simulink model "Australian14gen_forming_inertia"  (R2017b)
settings: Solver=ode23tb  StartTime=0.0  StopTime=100  FixedStep=1e-3  RelTol=1e-3  AbsTol=1e-3  EnableMultiTasking=on
PreLoadFcn:
  | dataaustralian14gen
values from neighbouring files (symbols this model uses):
  bus_v = [ 101	15 ... (first row only)    [dataaustralian14gen.m]
  c_fil = 1e-5*ones(15,1)    [dataaustralian14gen.m]
  comp = [ 1	211	0	0 ... (first row only)    [dataaustralian14gen.m]
  dist = sys.follin.dist    [main_following.m]    (also in main_forming.m = sys.formin.dist)
  Exc = [ 101	0	 200	0.1	    13.25  2.5	 0	0       0       0       0       0 ... (first row only)    [dataaustralian14gen.m]
  FH = 13    [dataaustralian14gen.m]
  FI = 1    [dataaustralian14gen.m]
  FL = .1    (= 0.1)    [dataaustralian14gen.m]
  G_data = [ 101	333.3	15	3.6	0.14	1.1	0.65	0.25	8.5     0.25	0.05	0       0       0.25	0.2 	0 ... (first row only)    [dataaustralian14gen.m]
  KH = 120    [dataaustralian14gen.m]
  KI = 10    [dataaustralian14gen.m]
  KL = 10    [dataaustralian14gen.m]
  Kvsc = 0*Kvsc    [dataaustralian14gen.m]    (also in optimgains.mat = [-4.89904313526 -21.043852985 -7.4754770322 -20.8245159401 -)
  l_fil = 5e-3*ones(15,1)    [dataaustralian14gen.m]
  line = [ 102	217	0.0084	0.0667	0.817	330	1 ... (first row only)    [dataaustralian14gen.m]
  load_mag = load_case4    [dataaustralian14gen.m]
  p = p_case4    [dataaustralian14gen.m]
  Pinit = [0.405553120017514,0.262363656270440,0.245287066765904,0.511573619715646,0.238910511748616,0.266289198874107,0.405451933295266,0.301363467877759,0.299904641553078,0.238601214125575,0.201576196829353,0.166515071179716,0.281316548159335,0.249279775700722,0.436119451429005]    [dataaustralian14gen.m]
  PSSMODEL = 1    [dataaustralian14gen.m]
  r_fil = 5e-1*ones(15,1)    [dataaustralian14gen.m]
  trans = [ 1	101	102	15	330	333.3	12	12 ... (first row only)    [dataaustralian14gen.m]
undefined symbols (not defined in the file or in its folder): D1, Delta, sys, thetavsc0
libraries: powerlib x399, Library x15, sps_avr x10, powerlib_extras x5
(part 4 of 4)

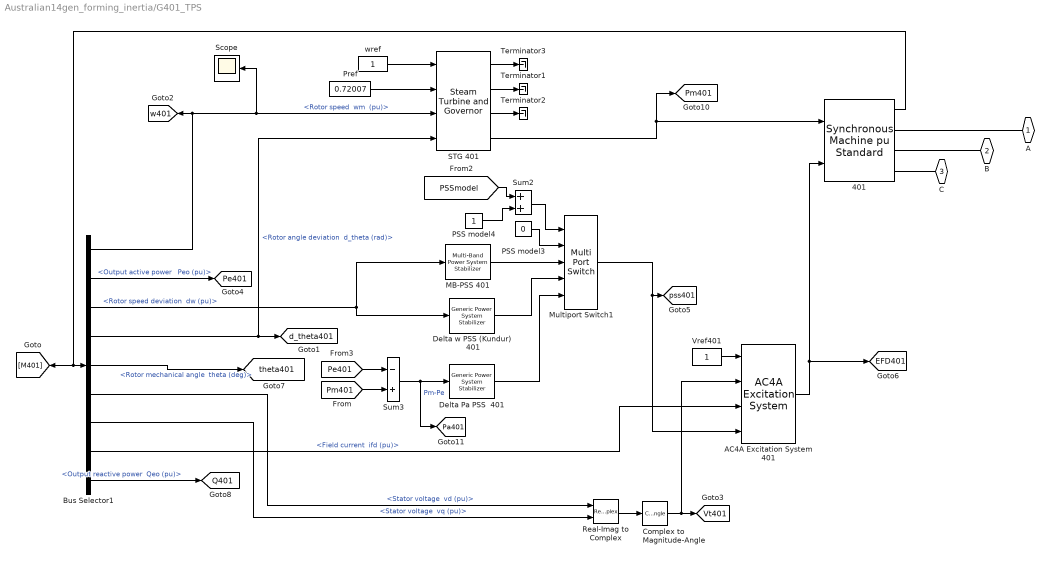
== system Australian14gen_forming_inertia/G401_TPS ==
  401 : powerlib/Machines/Synchronous Machine pu Standard  PresetModel=No  MechanicalLoad=Mechanical power Pm  ShowDetailedParameters=on  RotorType=Round  Units=per unit standard parameters  MeasurementBus=off  NominalParameters="[G_data(8,2)*1E6  G_data(8,3)*1E3  50]"  Reactances1=[G_data(8,6),G_data(8,8),G_data(8,10),G_data(8,7),G_data(8,12),G_data(8,14),G_data(8,5)]  Reactances2=[G_data(8,6),G_data(8,8),G_data(8,10),G_data(8,7),G_data(8,14),G_data(8,5)]  dAxisTimeConstants=Open-circuit  qAxisTimeConstants=Open-circuit  TimeConstants1="[G_data(8,9)  G_data(8,11)  G_data(8,15)]"  TimeConstants2="[G_data(8,9)  G_data(8,11)  G_data(8,13)  G_data(8,15)]"  TimeConstants3="[  5.9  0.033  0.023  ]"  TimeConstants4=[ 8.0, 0.03, 0.3371, 0.0295 ]  TimeConstants5=[ 1.01, 0.053, 0.1 ]  TimeConstants6=[ 1.3201, 0.023, 1.0, 0.07 ]  TimeConstants7="[  1.01  0.053  0.051266  ]"  TimeConstants8=[ 1.3201, 0.0231, 0.3371, 0.0295 ]  StatorResistance=0  Mechanical="[ G_data(8,4) 0  4 ]"  PolePairs=4  InitialConditions=[0 -57.8039 0.721852 0.721852 0.721852 -17.036 -137.036 102.964 1.85565]  SetSaturation=off  Saturation=[0.6404,0.7127,0.8441,0.9214,0.9956,1.082,1.19,1.316,1.457;0.7,0.7698,0.8872,0.9466,0.9969,1.046,1.1,1.151,1.201]  LoadFlowParameters=[1 960000000 20000 0 0]  TsPowergui=0  TsBlock=-1  IterativeModel=Forward Euler  IterativeDiscreteModel=Trapezoidal non iterative  BusType=PV  Pref=p(8,3)*1e6  Qref=0  Qmin=-inf  Qmax=inf  PLF=0  QLF=0
      settings: SourceProductName=Simscape Power Systems
  AC4A Excitation System 401 : sps_avr/AC4A Excitation System  Tr=Exc(8,2)  KaTa="[Exc(8,3)   Exc(8,4)]"  VIminmax=[-10 10]  VRminmax=[-4.53 5.64]  TbTc="[Exc(8,5)  Exc(8,6)]"  Kc=0  v0=[1 1.8556]  TsBlock=0
      settings: SourceProductName=Simscape Power Systems  SourceProductBaseCode=PS
  Bus Selector1 : BusSelector  OutputSignals="Mechanical.Rotor speed  wm  (pu),Output active power   Peo (pu),Mechanical.Rotor speed deviation  dw (pu),Mechanical.Rotor angle deviation  d_theta (rad),Mechanical.Rotor mechanical angle  theta (deg),dq0 components.Stator voltage  vd (pu),dq0 components.Stator voltage  vq (pu),dq0 components.Field current  ifd (pu),Output reactive power  Qeo (pu)"
  Complex to Magnitude-Angle : ComplexToMagnitudeAngle  Output=Magnitude
  Delta Pa PSS  401 : powerlib/Machines/Generic Power System Stabilizer  Tsensor=15e-3  K=2.5*1.25  Twashout=1  Tleadlag1=[60e-3 1]  Tleadlag2=[0 0]  VSlimits=[-0.15 0.15]  Vinit=0  Plot_On=off  MagdB_On=on  FreqRange=logspace(-2,2,500)
      settings: SourceProductName=Simscape Power Systems  SourceProductBaseCode=PS
  Delta w PSS (Kundur)  401 : powerlib/Machines/Generic Power System Stabilizer  Tsensor=15e-3  K=30  Twashout=10  Tleadlag1=[50e-3 20e-3]  Tleadlag2=[3 5.4]  VSlimits=[-0.15 0.15]  Vinit=0  Plot_On=off  MagdB_On=on  FreqRange=logspace(-2,2,500)
      settings: SourceProductName=Simscape Power Systems  SourceProductBaseCode=PS
  "MB-PSS 401 " : powerlib/Machines/Multi-Band Power System Stabilizer  OperationMode=Simplified settings  Kg=G  GL="[FL  KL]"  GI="[FI  KI]"  GH="[FH  KH]"  GLd=[66 66 9.4]  TcLF=[1.667 2 0 0 0 0 2 2.4 0 0 0 0 1 1]  GId=[66 66 47.6]  TcIF=[1 1 0.25 0.3 0 0 1 1 0.3 0.36 0 0 0 0]  GHd=[66 66 233]  TcHF="[0.01 0.012 0 0 0 0  0.012 0.0144 0 0 0 0 1 1]"  LIM=[.075 .15 .15 .15]  Plot_On=off  MagdB_On=off  FreqRange=logspace(-2,2,500)
      settings: SourceProductName=Simscape Power Systems  SourceProductBaseCode=PS
  Multiport Switch1 : MultiPortSwitch  Inputs=4  InputSameDT=on
  PSS model3 : Constant  Value=0
  PSS model4 : Constant
  Pref : Constant  Value=0.72007
  Real-Imag to Complex : RealImagToComplex
  STG 401 : powerlib/Machines/Steam Turbine and Governor  gentype=Tandem-compound (single mass)  reg1="[ 1  0.05    0 ]"  reg2="[ 0.001  0.15 ]"  reg3="[ -0.1  0.1  0  4.496 ]"  N=3000  turb1="[ 0  10   3.3   0.5   ]"  turb2="[   0   0.36    0.36   0.28   ]"  HA="[ 0.046  1.430  1.465   0.192 ]"  KA="[ 90.44  53.88  64.59   62.94  ]"  DA="[ 0.0115  0.3575  0.3663   0.0137  ]"  ini1=0.72007  ini2=[0.779316,-31.4247]
      settings: SourceProductName=Simscape Power Systems  SourceProductBaseCode=PS
  Scope : Scope
  Sum2 : Sum  SaturateOnIntegerOverflow=on  InputSameDT=on  OutDataTypeStr=Inherit: Same as first input
  Sum3 : Sum  Inputs=-+  SaturateOnIntegerOverflow=on  InputSameDT=on  OutDataTypeStr=Inherit: Same as first input
  Terminator1 : Terminator
  Terminator2 : Terminator
  Terminator3 : Terminator
  Vref401 : Constant
  wref : Constant
  A : PMIOPort  Port=1  Side=Left
  B : PMIOPort  Port=2  Side=Left
  C : PMIOPort  Port=3  Side=Left
  tag scope: EFD401=global, Pa401=global, Pe401=global, Pm401=global, Q401=global, Vt401=global, d_theta401=global, pss401=global, theta401=global, w401=global
  wires:
  Bus Selector1/7 -> Real-Imag to Complex/2  "<Stator voltage  vq (pu)>"
  Bus Selector1/6 -> Real-Imag to Complex/1  "<Stator voltage  vd (pu)>"
  wref/1 -> STG 401/1
  Vref401/1 -> AC4A Excitation System 401/1
  Bus Selector1/4 -> STG 401/4, [d_theta401]  "<Rotor angle deviation  d_theta (rad)>"
  401/1 -> [M401], Bus Selector1/1
  Bus Selector1/1 -> [w401], Scope/1, STG 401/3  "<Rotor speed  wm  (pu)>"
  Bus Selector1/3 -> Delta w PSS (Kundur)  401/1, "MB-PSS 401 "/1  "<Rotor speed deviation  dw (pu)>"
  Real-Imag to Complex/1 -> Complex to Magnitude-Angle/1
  Complex to Magnitude-Angle/1 -> AC4A Excitation System 401/2, [Vt401]
  AC4A Excitation System 401/1 -> 401/2, [EFD401]
  Multiport Switch1/1 -> AC4A Excitation System 401/4, [pss401]
  Bus Selector1/5 -> [theta401]  "<Rotor mechanical angle  theta (deg)>"
  Bus Selector1/2 -> [Pe401]  "<Output active power   Peo (pu)>"
  Bus Selector1/8 -> AC4A Excitation System 401/3  "<Field current  ifd (pu)>"
  STG 401/4 -> [Pm401], 401/1
  Pref/1 -> STG 401/2
  Bus Selector1/9 -> [Q401]  "<Output reactive power  Qeo (pu)>"
  PSS model4/1 -> Sum2/2
  Sum2/1 -> Multiport Switch1/1
  [PSSmodel] -> Sum2/1
  PSS model3/1 -> Multiport Switch1/2
  Sum3/1 -> [Pa401], Delta Pa PSS  401/1  "Pm-Pe"
  Delta Pa PSS  401/1 -> Multiport Switch1/5
  Delta w PSS (Kundur)  401/1 -> Multiport Switch1/4
  [Pm401] -> Sum3/2
  [Pe401] -> Sum3/1
  "MB-PSS 401 "/1 -> Multiport Switch1/3
  STG 401/1 -> Terminator3/1
  STG 401/2 -> Terminator1/1
  STG 401/3 -> Terminator2/1
  connections:
  401/RConn1 -- A/RConn1
  401/RConn2 -- B/RConn1
  401/RConn3 -- C/RConn1

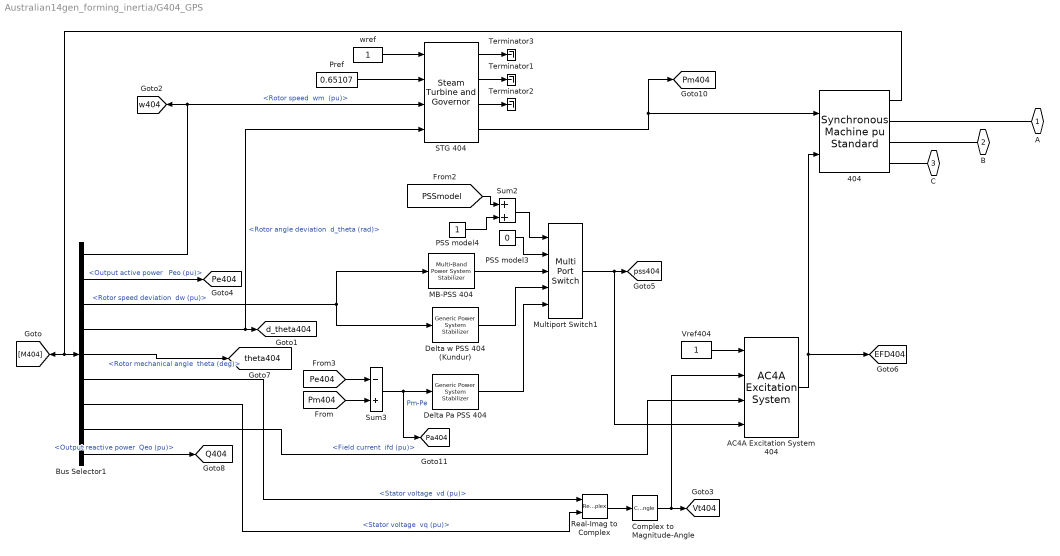
== system Australian14gen_forming_inertia/G404_GPS ==
  404 : powerlib/Machines/Synchronous Machine pu Standard  PresetModel=No  MechanicalLoad=Mechanical power Pm  ShowDetailedParameters=on  RotorType=Round  Units=per unit standard parameters  MeasurementBus=off  NominalParameters="[G_data(11,2)*1e6  G_data(11,3)*1e3  50]"  Reactances1="[G_data(11,6),G_data(11,8),G_data(11,10),G_data(11,7),  G_data(11,12),G_data(11,14),G_data(11,5)]"  Reactances2="[G_data(11,6),G_data(11,8),G_data(11,10),G_data(11,7),  G_data(11,12),G_data(11,14),G_data(11,5)]"  dAxisTimeConstants=Open-circuit  qAxisTimeConstants=Open-circuit  TimeConstants1="[G_data(11,9)  G_data(11,11)   G_data(11,13) G_data(11,15)]"  TimeConstants2="[G_data(11,9)  G_data(11,11)   G_data(11,13)  G_data(11,15)]"  TimeConstants3="[  5.9  0.033  0.023  ]"  TimeConstants4=[ 8.0, 0.03, 0.3371, 0.0295 ]  TimeConstants5=[ 1.01, 0.053, 0.1 ]  TimeConstants6=[ 1.3201, 0.023, 1.0, 0.07 ]  TimeConstants7="[  1.01  0.053  0.051266  ]"  TimeConstants8=[ 1.3201, 0.0231, 0.3371, 0.0295 ]  StatorResistance=0  Mechanical="[ G_data(11,4) 0  4 ]"  PolePairs=4  InitialConditions=[0 -60.4485 0.651109 0.651109 0.651109 -12.436 -132.436 107.564 1.69373]  SetSaturation=off  Saturation=[0.6404,0.7127,0.8441,0.9214,0.9956,1.082,1.19,1.316,1.457;0.7,0.7698,0.8872,0.9466,0.9969,1.046,1.1,1.151,1.201]  LoadFlowParameters=[1 651000000 20000 0 0]  TsPowergui=0  TsBlock=-1  IterativeModel=Forward Euler  IterativeDiscreteModel=Trapezoidal non iterative  BusType=PV  Pref=p(11,3)*1e6  Qref=0  Qmin=-inf  Qmax=inf  PLF=0  QLF=0
      settings: SourceProductName=Simscape Power Systems
  AC4A Excitation System 404 : sps_avr/AC4A Excitation System  Tr=Exc(11,2)  KaTa="[Exc(11,3)   Exc(11,4)]"  VIminmax=[-10 10]  VRminmax=[-4.53 5.64]  TbTc="[Exc(11,5)  Exc(11,6)]"  Kc=0  v0=[1 1.6937]  TsBlock=0
      settings: SourceProductName=Simscape Power Systems  SourceProductBaseCode=PS
  Bus Selector1 : BusSelector  OutputSignals="Mechanical.Rotor speed  wm  (pu),Output active power   Peo (pu),Mechanical.Rotor speed deviation  dw (pu),Mechanical.Rotor angle deviation  d_theta (rad),Mechanical.Rotor mechanical angle  theta (deg),dq0 components.Stator voltage  vd (pu),dq0 components.Stator voltage  vq (pu),dq0 components.Field current  ifd (pu),Output reactive power  Qeo (pu)"
  Complex to Magnitude-Angle : ComplexToMagnitudeAngle  Output=Magnitude
  "Delta Pa PSS 404 " : powerlib/Machines/Generic Power System Stabilizer  Tsensor=15e-3  K=2.5*1.25  Twashout=1  Tleadlag1=[60e-3 1]  Tleadlag2=[0 0]  VSlimits=[-0.15 0.15]  Vinit=0  Plot_On=off  MagdB_On=on  FreqRange=logspace(-2,2,500)
      settings: SourceProductName=Simscape Power Systems  SourceProductBaseCode=PS
  "Delta w PSS 404 (Kundur) " : powerlib/Machines/Generic Power System Stabilizer  Tsensor=15e-3  K=30  Twashout=10  Tleadlag1=[50e-3 20e-3]  Tleadlag2=[3 5.4]  VSlimits=[-0.15 0.15]  Vinit=0  Plot_On=off  MagdB_On=on  FreqRange=logspace(-2,2,500)
      settings: SourceProductName=Simscape Power Systems  SourceProductBaseCode=PS
  "MB-PSS 404 " : powerlib/Machines/Multi-Band Power System Stabilizer  OperationMode=Simplified settings  Kg=G  GL="[FL  KL]"  GI="[FI  KI]"  GH="[FH  KH]"  GLd=[66 66 9.4]  TcLF=[1.667 2 0 0 0 0 2 2.4 0 0 0 0 1 1]  GId=[66 66 47.6]  TcIF=[1 1 0.25 0.3 0 0 1 1 0.3 0.36 0 0 0 0]  GHd=[66 66 233]  TcHF="[0.01 0.012 0 0 0 0  0.012 0.0144 0 0 0 0 1 1]"  LIM=[.075 .15 .15 .15]  Plot_On=off  MagdB_On=off  FreqRange=logspace(-2,2,500)
      settings: SourceProductName=Simscape Power Systems  SourceProductBaseCode=PS
  Multiport Switch1 : MultiPortSwitch  Inputs=4  InputSameDT=on
  PSS model3 : Constant  Value=0
  PSS model4 : Constant
  Pref : Constant  Value=0.65107
  Real-Imag to Complex : RealImagToComplex
  STG 404 : powerlib/Machines/Steam Turbine and Governor  gentype=Tandem-compound (single mass)  reg1="[ 1  0.05    0 ]"  reg2="[ 0.001  0.15 ]"  reg3="[ -0.1  0.1  0  4.496 ]"  N=3000  turb1="[ 0  10   3.3   0.5   ]"  turb2="[   0   0.36    0.36   0.28   ]"  HA="[ 0.046  1.430  1.465   0.192 ]"  KA="[ 90.44  53.88  64.59   62.94  ]"  DA="[ 0.0115  0.3575  0.3663   0.0137  ]"  ini1=0.65107  ini2=[0.779316,-31.4247]
      settings: SourceProductName=Simscape Power Systems  SourceProductBaseCode=PS
  Sum2 : Sum  SaturateOnIntegerOverflow=on  InputSameDT=on  OutDataTypeStr=Inherit: Same as first input
  Sum3 : Sum  Inputs=-+  SaturateOnIntegerOverflow=on  InputSameDT=on  OutDataTypeStr=Inherit: Same as first input
  Terminator1 : Terminator
  Terminator2 : Terminator
  Terminator3 : Terminator
  Vref404 : Constant
  wref : Constant
  A : PMIOPort  Port=1  Side=Left
  B : PMIOPort  Port=2  Side=Left
  C : PMIOPort  Port=3  Side=Left
  tag scope: EFD404=global, Pa404=global, Pe404=global, Pm404=global, Q404=global, Vt404=global, d_theta404=global, pss404=global, theta404=global, w404=global
  wires:
  Bus Selector1/7 -> Real-Imag to Complex/2  "<Stator voltage  vq (pu)>"
  Bus Selector1/6 -> Real-Imag to Complex/1  "<Stator voltage  vd (pu)>"
  wref/1 -> STG 404/1
  Vref404/1 -> AC4A Excitation System 404/1
  Bus Selector1/4 -> STG 404/4, [d_theta404]  "<Rotor angle deviation  d_theta (rad)>"
  404/1 -> [M404], Bus Selector1/1
  Bus Selector1/1 -> [w404], STG 404/3  "<Rotor speed  wm  (pu)>"
  Bus Selector1/3 -> "MB-PSS 404 "/1, "Delta w PSS 404 (Kundur) "/1  "<Rotor speed deviation  dw (pu)>"
  Real-Imag to Complex/1 -> Complex to Magnitude-Angle/1
  Complex to Magnitude-Angle/1 -> AC4A Excitation System 404/2, [Vt404]
  AC4A Excitation System 404/1 -> 404/2, [EFD404]
  Multiport Switch1/1 -> AC4A Excitation System 404/4, [pss404]
  Bus Selector1/5 -> [theta404]  "<Rotor mechanical angle  theta (deg)>"
  Bus Selector1/2 -> [Pe404]  "<Output active power   Peo (pu)>"
  Bus Selector1/8 -> AC4A Excitation System 404/3  "<Field current  ifd (pu)>"
  Pref/1 -> STG 404/2
  STG 404/4 -> [Pm404], 404/1
  Bus Selector1/9 -> [Q404]  "<Output reactive power  Qeo (pu)>"
  PSS model4/1 -> Sum2/2
  Sum2/1 -> Multiport Switch1/1
  [PSSmodel] -> Sum2/1
  PSS model3/1 -> Multiport Switch1/2
  Sum3/1 -> [Pa404], "Delta Pa PSS 404 "/1  "Pm-Pe"
  "Delta Pa PSS 404 "/1 -> Multiport Switch1/5
  "Delta w PSS 404 (Kundur) "/1 -> Multiport Switch1/4
  [Pm404] -> Sum3/2
  [Pe404] -> Sum3/1
  "MB-PSS 404 "/1 -> Multiport Switch1/3
  STG 404/1 -> Terminator3/1
  STG 404/2 -> Terminator1/1
  STG 404/3 -> Terminator2/1
  connections:
  404/RConn1 -- A/RConn1
  404/RConn2 -- B/RConn1
  404/RConn3 -- C/RConn1

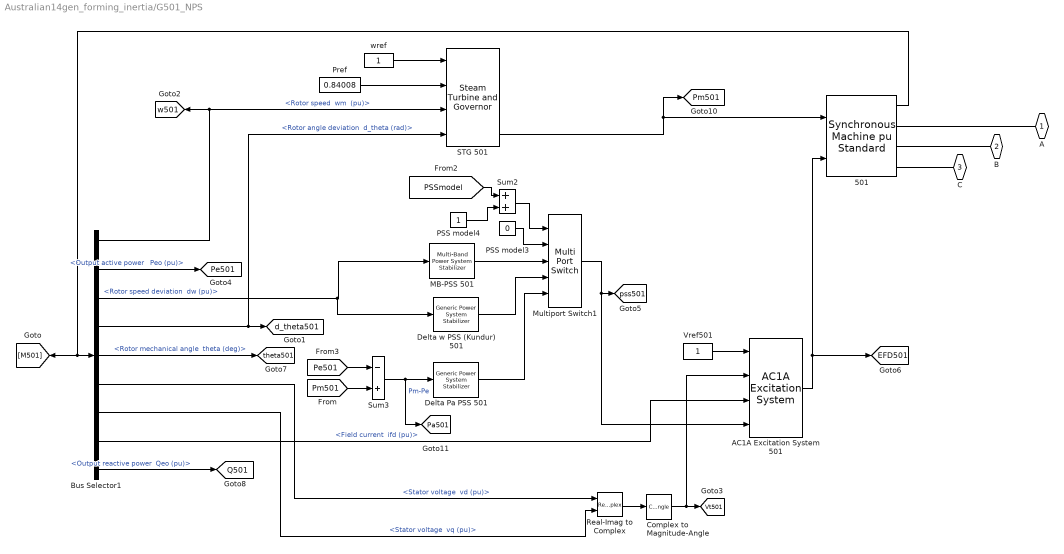
== system Australian14gen_forming_inertia/G501_NPS ==
  501 : powerlib/Machines/Synchronous Machine pu Standard  PresetModel=No  MechanicalLoad=Mechanical power Pm  ShowDetailedParameters=on  RotorType=Round  Units=per unit standard parameters  MeasurementBus=off  NominalParameters="[G_data(12,2)*1E6  G_data(12,3)*1E3  50]"  Reactances1=[G_data(12,6),G_data(12,8),G_data(12,10),G_data(12,7),G_data(12,12),G_data(12,14),G_data(12,5)]  Reactances2=[G_data(12,6),G_data(12,8),G_data(12,10),G_data(12,7),G_data(12,12),G_data(12,14),G_data(12,5)]  dAxisTimeConstants=Open-circuit  qAxisTimeConstants=Open-circuit  TimeConstants1="[G_data(12,9)  G_data(12,11)  G_data(12,13) G_data(12,15)]"  TimeConstants2="[G_data(12,9)  G_data(12,11)  G_data(12,13) G_data(12,15)]"  TimeConstants3="[  5.9  0.033  0.023  ]"  TimeConstants4=[ 8.0, 0.03, 0.3371, 0.0295 ]  TimeConstants5=[ 1.01, 0.053, 0.1 ]  TimeConstants6=[ 1.3201, 0.023, 1.0, 0.07 ]  TimeConstants7="[  1.01  0.053  0.051266  ]"  TimeConstants8=[ 1.3201, 0.0231, 0.3371, 0.0295 ]  StatorResistance=0  Mechanical="[ G_data(12,4) 0  4 ]"  PolePairs=4  InitialConditions=[0 -60.6578 0.858474 0.858474 0.858474 -22.6802 -142.68 97.3198 1.92862]  SetSaturation=off  Saturation=[0.6404,0.7127,0.8441,0.9214,0.9956,1.082,1.19,1.316,1.457;0.7,0.7698,0.8872,0.9466,0.9969,1.046,1.1,1.151,1.201]  LoadFlowParameters=[1 560000000 20000 0 0]  TsPowergui=0  TsBlock=-1  IterativeModel=Forward Euler  IterativeDiscreteModel=Trapezoidal non iterative  BusType=PV  Pref=p(12,3)*1e6  Qref=0  Qmin=-inf  Qmax=inf  PLF=0  QLF=0
      settings: SourceProductName=Simscape Power Systems
  AC1A Excitation System 501 : sps_avr/AC1A Excitation System  Tr=Exc(12,2)  KaTa="[Exc(12,3)   Exc(12,4)]"  VAminmax=[-14.5 14.5]  VRminmax=[-5.43 6.03]  KfTf="[Exc(12,9)  Exc(12,10)]"  TbTc="[Exc(12,5)  Exc(12,6)]"  KeTe="[Exc(12,7)  Exc(12,8)]"  Ve12=[4.18 3.14]  SeVe12=[0.10 0.03]  Kd=0.38  Kc=0.20  v0=[1 1.9286]  TsBlock=0
      settings: SourceProductName=Simscape Power Systems  SourceProductBaseCode=PS
  Bus Selector1 : BusSelector  OutputSignals="Mechanical.Rotor speed  wm  (pu),Output active power   Peo (pu),Mechanical.Rotor speed deviation  dw (pu),Mechanical.Rotor angle deviation  d_theta (rad),Mechanical.Rotor mechanical angle  theta (deg),dq0 components.Stator voltage  vd (pu),dq0 components.Stator voltage  vq (pu),dq0 components.Field current  ifd (pu),Output reactive power  Qeo (pu)"
  Complex to Magnitude-Angle : ComplexToMagnitudeAngle  Output=Magnitude
  "Delta Pa PSS 501 " : powerlib/Machines/Generic Power System Stabilizer  Tsensor=15e-3  K=2.5*1.25  Twashout=1  Tleadlag1=[60e-3 1]  Tleadlag2=[0 0]  VSlimits=[-0.15 0.15]  Vinit=0  Plot_On=off  MagdB_On=on  FreqRange=logspace(-2,2,500)
      settings: SourceProductName=Simscape Power Systems  SourceProductBaseCode=PS
  "Delta w PSS (Kundur) 501 " : powerlib/Machines/Generic Power System Stabilizer  Tsensor=15e-3  K=30  Twashout=10  Tleadlag1=[50e-3 20e-3]  Tleadlag2=[3 5.4]  VSlimits=[-0.15 0.15]  Vinit=0  Plot_On=off  MagdB_On=on  FreqRange=logspace(-2,2,500)
      settings: SourceProductName=Simscape Power Systems  SourceProductBaseCode=PS
  "MB-PSS 501 " : powerlib/Machines/Multi-Band Power System Stabilizer  OperationMode=Simplified settings  Kg=G  GL="[FL  KL]"  GI="[FI  KI]"  GH="[FH  KH]"  GLd=[66 66 9.4]  TcLF=[1.667 2 0 0 0 0 2 2.4 0 0 0 0 1 1]  GId=[66 66 47.6]  TcIF=[1 1 0.25 0.3 0 0 1 1 0.3 0.36 0 0 0 0]  GHd=[66 66 233]  TcHF="[0.01 0.012 0 0 0 0  0.012 0.0144 0 0 0 0 1 1]"  LIM=[.075 .15 .15 .15]  Plot_On=off  MagdB_On=off  FreqRange=logspace(-2,2,500)
      settings: SourceProductName=Simscape Power Systems  SourceProductBaseCode=PS
  Multiport Switch1 : MultiPortSwitch  Inputs=4  InputSameDT=on
  PSS model3 : Constant  Value=0
  PSS model4 : Constant
  Pref : Constant  Value=0.84008
  Real-Imag to Complex : RealImagToComplex
  STG 501 : powerlib/Machines/Steam Turbine and Governor  gentype=Tandem-compound (single mass)  reg1="[ 1  0.05    0 ]"  reg2="[ 0.001  0.15 ]"  reg3="[ -0.1  0.1  0  4.496 ]"  N=3000  turb1="[ 0  10   3.3   0.5   ]"  turb2="[   0   0.36    0.36   0.28   ]"  HA="[ 0.046  1.430  1.465   0.192 ]"  KA="[ 90.44  53.88  64.59   62.94  ]"  DA="[ 0.0115  0.3575  0.3663   0.0137  ]"  ini1=0.84008  ini2=[0.779316,-31.4247]
      settings: SourceProductName=Simscape Power Systems  SourceProductBaseCode=PS
  Sum2 : Sum  SaturateOnIntegerOverflow=on  InputSameDT=on  OutDataTypeStr=Inherit: Same as first input
  Sum3 : Sum  Inputs=-+  SaturateOnIntegerOverflow=on  InputSameDT=on  OutDataTypeStr=Inherit: Same as first input
  Vref501 : Constant
  wref : Constant
  A : PMIOPort  Port=1  Side=Left
  B : PMIOPort  Port=2  Side=Left
  C : PMIOPort  Port=3  Side=Left
  tag scope: EFD501=global, Pa501=global, Pe501=global, Pm501=global, Q501=global, Vt501=global, d_theta501=global, pss501=global, theta501=global, w501=global
  wires:
  Bus Selector1/7 -> Real-Imag to Complex/2  "<Stator voltage  vq (pu)>"
  Bus Selector1/6 -> Real-Imag to Complex/1  "<Stator voltage  vd (pu)>"
  wref/1 -> STG 501/1
  Vref501/1 -> AC1A Excitation System 501/1
  Bus Selector1/4 -> STG 501/4, [d_theta501]  "<Rotor angle deviation  d_theta (rad)>"
  501/1 -> [M501], Bus Selector1/1
  Bus Selector1/1 -> [w501], STG 501/3  "<Rotor speed  wm  (pu)>"
  Bus Selector1/3 -> "Delta w PSS (Kundur) 501 "/1, "MB-PSS 501 "/1  "<Rotor speed deviation  dw (pu)>"
  Real-Imag to Complex/1 -> Complex to Magnitude-Angle/1
  Complex to Magnitude-Angle/1 -> AC1A Excitation System 501/2, [Vt501]
  AC1A Excitation System 501/1 -> 501/2, [EFD501]
  Multiport Switch1/1 -> AC1A Excitation System 501/4, [pss501]
  Bus Selector1/5 -> [theta501]  "<Rotor mechanical angle  theta (deg)>"
  Bus Selector1/2 -> [Pe501]  "<Output active power   Peo (pu)>"
  Bus Selector1/8 -> AC1A Excitation System 501/3  "<Field current  ifd (pu)>"
  STG 501/4 -> [Pm501], 501/1
  Pref/1 -> STG 501/2
  Bus Selector1/9 -> [Q501]  "<Output reactive power  Qeo (pu)>"
  PSS model4/1 -> Sum2/2
  Sum2/1 -> Multiport Switch1/1
  [PSSmodel] -> Sum2/1
  PSS model3/1 -> Multiport Switch1/2
  Sum3/1 -> [Pa501], "Delta Pa PSS 501 "/1  "Pm-Pe"
  "Delta Pa PSS 501 "/1 -> Multiport Switch1/5
  "Delta w PSS (Kundur) 501 "/1 -> Multiport Switch1/4
  [Pm501] -> Sum3/2
  [Pe501] -> Sum3/1
  "MB-PSS 501 "/1 -> Multiport Switch1/3
  connections:
  501/RConn1 -- A/RConn1
  501/RConn2 -- B/RConn1
  501/RConn3 -- C/RConn1

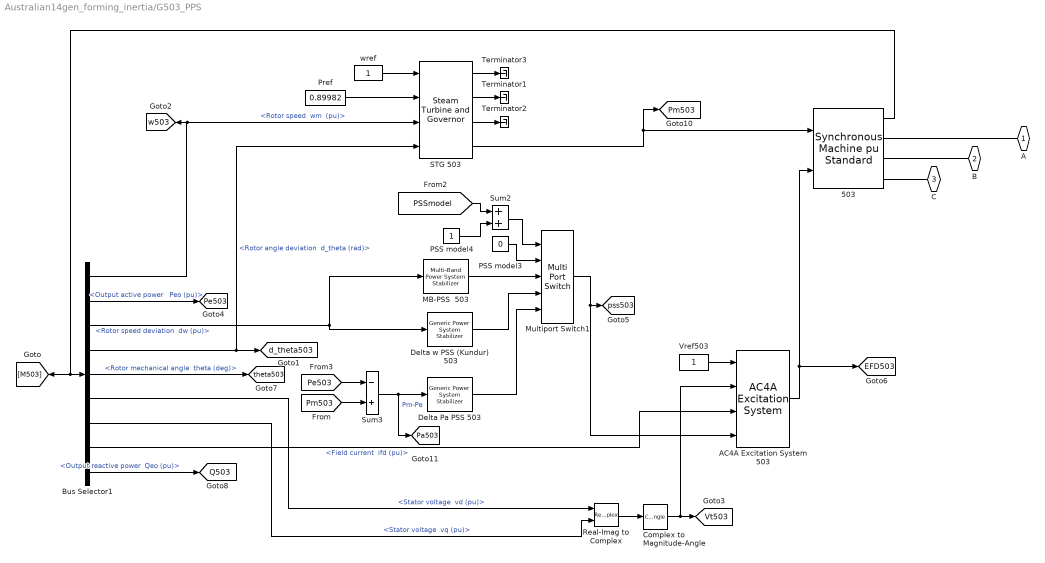
== system Australian14gen_forming_inertia/G503_PPS ==
  503 : powerlib/Machines/Synchronous Machine pu Standard  PresetModel=No  MechanicalLoad=Mechanical power Pm  ShowDetailedParameters=on  RotorType=Round  Units=per unit standard parameters  MeasurementBus=off  NominalParameters="[G_data(14,2)*1E6  G_data(14,3)*1E3  50]"  Reactances1=[G_data(14,6),G_data(14,8),G_data(14,10),G_data(14,7),G_data(14,12),G_data(14,14),G_data(14,5)]  Reactances2=[G_data(14,6),G_data(14,8),G_data(14,10),G_data(14,7),G_data(14,12),G_data(14,14),G_data(14,5)]  dAxisTimeConstants=Open-circuit  qAxisTimeConstants=Open-circuit  TimeConstants1="[G_data(14,9)  G_data(14,11) G_data(14,13)  G_data(14,15)]"  TimeConstants2="[G_data(14,9)  G_data(14,11) G_data(14,13)  G_data(14,15)]"  TimeConstants3="[  5.9  0.033  0.023  ]"  TimeConstants4=[ 8.0, 0.03, 0.3371, 0.0295 ]  TimeConstants5=[ 1.01, 0.053, 0.1 ]  TimeConstants6=[ 1.3201, 0.023, 1.0, 0.07 ]  TimeConstants7="[  1.01  0.053  0.051266  ]"  TimeConstants8=[ 1.3201, 0.0231, 0.3371, 0.0295 ]  StatorResistance=0  Mechanical=[ G_data(14,4) 0 4 ]  PolePairs=4  InitialConditions=[0 -63.1155 0.904039 0.904039 0.904039 -32.9362 -152.936 87.0638 2.2144]  SetSaturation=off  Saturation=[0.6404,0.7127,0.8441,0.9214,0.9956,1.082,1.19,1.316,1.457;0.7,0.7698,0.8872,0.9466,0.9969,1.046,1.1,1.151,1.201]  LoadFlowParameters=[1 150000000 15000 0 0]  TsPowergui=0  TsBlock=-1  IterativeModel=Forward Euler  IterativeDiscreteModel=Trapezoidal non iterative  BusType=PV  Pref=p(14,3)*1e6  Qref=0  Qmin=-inf  Qmax=inf  PLF=0  QLF=0
      settings: SourceProductName=Simscape Power Systems
  AC4A Excitation System 503 : sps_avr/AC4A Excitation System  Tr=Exc(14,2)  KaTa="[Exc(14,3)   Exc(14,4)]"  VIminmax=[-10 10]  VRminmax=[-4.53 5.64]  TbTc="[Exc(14,5)  Exc(14,6)]"  Kc=0  v0=[1 2.2144]  TsBlock=0
      settings: SourceProductName=Simscape Power Systems  SourceProductBaseCode=PS
  Bus Selector1 : BusSelector  OutputSignals="Mechanical.Rotor speed  wm  (pu),Output active power   Peo (pu),Mechanical.Rotor speed deviation  dw (pu),Mechanical.Rotor angle deviation  d_theta (rad),Mechanical.Rotor mechanical angle  theta (deg),dq0 components.Stator voltage  vd (pu),dq0 components.Stator voltage  vq (pu),dq0 components.Field current  ifd (pu),Output reactive power  Qeo (pu)"
  Complex to Magnitude-Angle : ComplexToMagnitudeAngle  Output=Magnitude
  "Delta Pa PSS 503 " : powerlib/Machines/Generic Power System Stabilizer  Tsensor=15e-3  K=2.5*1.25  Twashout=1  Tleadlag1=[60e-3 1]  Tleadlag2=[0 0]  VSlimits=[-0.15 0.15]  Vinit=0  Plot_On=off  MagdB_On=on  FreqRange=logspace(-2,2,500)
      settings: SourceProductName=Simscape Power Systems  SourceProductBaseCode=PS
  Delta w PSS (Kundur)  503 : powerlib/Machines/Generic Power System Stabilizer  Tsensor=15e-3  K=30  Twashout=10  Tleadlag1=[50e-3 20e-3]  Tleadlag2=[3 5.4]  VSlimits=[-0.15 0.15]  Vinit=0  Plot_On=off  MagdB_On=on  FreqRange=logspace(-2,2,500)
      settings: SourceProductName=Simscape Power Systems  SourceProductBaseCode=PS
  MB-PSS  503 : powerlib/Machines/Multi-Band Power System Stabilizer  OperationMode=Simplified settings  Kg=G  GL="[FL  KL]"  GI="[FI  KI]"  GH="[FH  KH]"  GLd=[66 66 9.4]  TcLF=[1.667 2 0 0 0 0 2 2.4 0 0 0 0 1 1]  GId=[66 66 47.6]  TcIF=[1 1 0.25 0.3 0 0 1 1 0.3 0.36 0 0 0 0]  GHd=[66 66 233]  TcHF="[0.01 0.012 0 0 0 0  0.012 0.0144 0 0 0 0 1 1]"  LIM=[.075 .15 .15 .15]  Plot_On=off  MagdB_On=off  FreqRange=logspace(-2,2,500)
      settings: SourceProductName=Simscape Power Systems  SourceProductBaseCode=PS
  Multiport Switch1 : MultiPortSwitch  Inputs=4  InputSameDT=on
  PSS model3 : Constant  Value=0
  PSS model4 : Constant
  Pref : Constant  Value=0.89982
  Real-Imag to Complex : RealImagToComplex
  STG 503 : powerlib/Machines/Steam Turbine and Governor  gentype=Tandem-compound (single mass)  reg1="[ 1  0.05    0 ]"  reg2="[ 0.001  0.15 ]"  reg3="[ -0.1  0.1  0  4.496 ]"  N=3000  turb1="[ 0  10   3.3   0.5   ]"  turb2="[   0   0.36    0.36   0.28   ]"  HA="[ 0.046  1.430  1.465   0.192 ]"  KA="[ 90.44  53.88  64.59   62.94  ]"  DA="[ 0.0115  0.3575  0.3663   0.0137  ]"  ini1=0.89982  ini2=[0.779316,-31.4247]
      settings: SourceProductName=Simscape Power Systems  SourceProductBaseCode=PS
  Sum2 : Sum  SaturateOnIntegerOverflow=on  InputSameDT=on  OutDataTypeStr=Inherit: Same as first input
  Sum3 : Sum  Inputs=-+  SaturateOnIntegerOverflow=on  InputSameDT=on  OutDataTypeStr=Inherit: Same as first input
  Terminator1 : Terminator
  Terminator2 : Terminator
  Terminator3 : Terminator
  Vref503 : Constant
  wref : Constant
  A : PMIOPort  Port=1  Side=Left
  B : PMIOPort  Port=2  Side=Left
  C : PMIOPort  Port=3  Side=Left
  tag scope: EFD503=global, Pa503=global, Pe503=global, Pm503=global, Q503=global, Vt503=global, d_theta503=global, pss503=global, theta503=global, w503=global
  wires:
  Bus Selector1/7 -> Real-Imag to Complex/2  "<Stator voltage  vq (pu)>"
  Bus Selector1/6 -> Real-Imag to Complex/1  "<Stator voltage  vd (pu)>"
  wref/1 -> STG 503/1
  Vref503/1 -> AC4A Excitation System 503/1
  Bus Selector1/4 -> STG 503/4, [d_theta503]  "<Rotor angle deviation  d_theta (rad)>"
  503/1 -> [M503], Bus Selector1/1
  Bus Selector1/1 -> [w503], STG 503/3  "<Rotor speed  wm  (pu)>"
  Bus Selector1/3 -> MB-PSS  503/1, Delta w PSS (Kundur)  503/1  "<Rotor speed deviation  dw (pu)>"
  Real-Imag to Complex/1 -> Complex to Magnitude-Angle/1
  Complex to Magnitude-Angle/1 -> AC4A Excitation System 503/2, [Vt503]
  AC4A Excitation System 503/1 -> 503/2, [EFD503]
  Multiport Switch1/1 -> AC4A Excitation System 503/4, [pss503]
  Bus Selector1/5 -> [theta503]  "<Rotor mechanical angle  theta (deg)>"
  Bus Selector1/2 -> [Pe503]  "<Output active power   Peo (pu)>"
  Bus Selector1/8 -> AC4A Excitation System 503/3  "<Field current  ifd (pu)>"
  Pref/1 -> STG 503/2
  STG 503/4 -> [Pm503], 503/1
  Bus Selector1/9 -> [Q503]  "<Output reactive power  Qeo (pu)>"
  PSS model4/1 -> Sum2/2
  Sum2/1 -> Multiport Switch1/1
  [PSSmodel] -> Sum2/1
  PSS model3/1 -> Multiport Switch1/2
  Sum3/1 -> [Pa503], "Delta Pa PSS 503 "/1  "Pm-Pe"
  "Delta Pa PSS 503 "/1 -> Multiport Switch1/5
  Delta w PSS (Kundur)  503/1 -> Multiport Switch1/4
  [Pm503] -> Sum3/2
  [Pe503] -> Sum3/1
  MB-PSS  503/1 -> Multiport Switch1/3
  STG 503/1 -> Terminator3/1
  STG 503/2 -> Terminator1/1
  STG 503/3 -> Terminator2/1
  connections:
  503/RConn1 -- A/RConn1
  503/RConn2 -- B/RConn1
  503/RConn3 -- C/RConn1

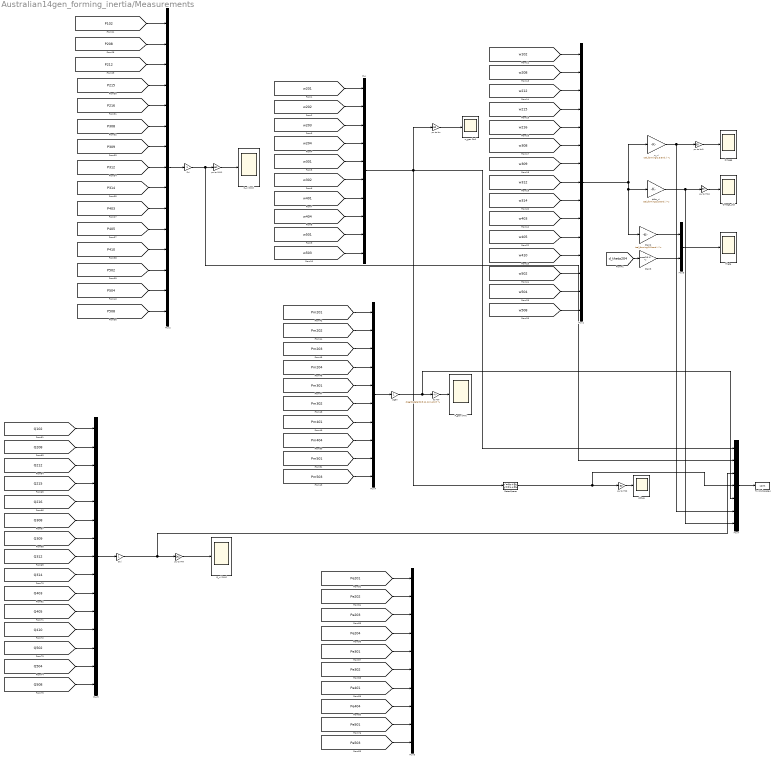
== system Australian14gen_forming_inertia/Measurements ==
  Gain2 : Gain  Gain=Isel_forming(3:3:end,:)  Multiplication=Matrix(K*u) (u vector)
  Gain3 : Gain  Gain=ones(15,1)  Multiplication=Matrix(K*u) (u vector)
  Mux : Mux  Inputs=10
  Mux1 : Mux  Inputs=15
  Mux2 : Mux  Inputs=15
  Mux3 : Mux  Inputs=2
  Mux4 : Mux  Inputs=10
  Mux5 : Mux  Inputs=15
  Mux6 : Mux  Inputs=10
  Mux7 : Mux  Inputs=7
  Omega : Scope
  Omega_dot : Scope
  P_gen [MW] : Scope
  P_vi [MW] : Scope
  Pvi : Gain
  Q_vi [MW] : Scope
  Qvi : Gain
  State-Space : StateSpace  A=sys.formin.filt.A  B=sys.formin.filt.B  C=sys.formin.filt.C  D=sys.formin.filt.D  InitialCondition=0
  Theta : Scope
  To Workspace4 : ToWorkspace  VariableName=ysim  SaveFormat=Timeseries  SampleTime=-1
  ddtw_vi : Gain  Gain=Isel_forming(2:3:end,:)  Multiplication=Matrix(K*u) (u vector)
  ddtwg : Scope
  pgen : Gain
  pu to Hz : Gain  Gain=50
  pu to Hz/s : Gain  Gain=50
  pu to Hz1 : Gain  Gain=50
  pu to Hz2 : Gain  Gain=50
  pu to MW : Gain  Gain=1e2
  pu to MW1 : Gain  Gain=1e2
  to MW : Gain  Gain=diag(G_data([2:8,11,12,14],2))  Multiplication=Matrix(K*u) (u vector)
  w_gen [Hz] : Scope
  w_vi : Gain  Gain=Isel_forming(1:3:end,:)  Multiplication=Matrix(K*u) (u vector)
  wires:
  [w201] -> Mux/1
  [w202] -> Mux/2
  [w203] -> Mux/3
  [w204] -> Mux/4
  [w301] -> Mux/5
  [w302] -> Mux/6
  [w401] -> Mux/7
  [w404] -> Mux/8
  [w501] -> Mux/9
  [w503] -> Mux/10
  [w312] -> Mux1/8
  [w403] -> Mux1/10
  [w314] -> Mux1/9
  [w208] -> Mux1/2
  [w309] -> Mux1/7
  [w308] -> Mux1/6
  [w215] -> Mux1/4
  [w212] -> Mux1/3
  [w102] -> Mux1/1
  [w216] -> Mux1/5
  [w502] -> Mux1/13
  [w504] -> Mux1/14
  [w508] -> Mux1/15
  [w410] -> Mux1/12
  [w405] -> Mux1/11
  w_vi/1 -> Mux7/6, pu to Hz1/1
  Mux1/1 -> w_vi/1, Gain2/1, ddtw_vi/1
  ddtw_vi/1 -> Mux7/7, pu to Hz/s/1
  [P212] -> Mux2/3
  [P312] -> Mux2/8
  [P309] -> Mux2/7
  [P208] -> Mux2/2
  Mux2/1 -> Pvi/1
  [P308] -> Mux2/6
  [P403] -> Mux2/10
  [P215] -> Mux2/4
  [P102] -> Mux2/1
  [P314] -> Mux2/9
  [P216] -> Mux2/5
  [P405] -> Mux2/11
  [P410] -> Mux2/12
  [P502] -> Mux2/13
  [P504] -> Mux2/14
  [P508] -> Mux2/15
  [d_theta204] -> Gain3/1
  Mux3/1 -> Theta/1
  [Pm404] -> Mux4/8
  [Pm401] -> Mux4/7
  [Pm204] -> Mux4/4
  [Pm501] -> Mux4/9
  [Pm302] -> Mux4/6
  [Pm201] -> Mux4/1
  [Pm503] -> Mux4/10
  [Pm202] -> Mux4/2
  Mux4/1 -> pgen/1
  [Pm301] -> Mux4/5
  [Pm203] -> Mux4/3
  [Q215] -> Mux5/4
  [Q309] -> Mux5/7
  [Q314] -> Mux5/9
  [Q208] -> Mux5/2
  Mux5/1 -> Qvi/1
  [Q102] -> Mux5/1
  [Q212] -> Mux5/3
  [Q504] -> Mux5/14
  [Q216] -> Mux5/5
  [Q312] -> Mux5/8
  [Q502] -> Mux5/13
  [Q308] -> Mux5/6
  [Q403] -> Mux5/10
  [Q508] -> Mux5/15
  [Q405] -> Mux5/11
  [Q410] -> Mux5/12
  [Pe302] -> Mux6/6
  [Pe203] -> Mux6/3
  [Pe204] -> Mux6/4
  [Pe201] -> Mux6/1
  [Pe404] -> Mux6/8
  [Pe202] -> Mux6/2
  [Pe503] -> Mux6/10
  [Pe501] -> Mux6/9
  [Pe401] -> Mux6/7
  [Pe301] -> Mux6/5
  pgen/1 -> Mux7/5, to MW/1
  Qvi/1 -> Mux7/3, pu to MW/1
  pu to MW/1 -> Q_vi [MW]/1
  Pvi/1 -> Mux7/2, pu to MW1/1
  pu to MW1/1 -> P_vi [MW]/1
  pu to Hz/1 -> w_gen [Hz]/1
  to MW/1 -> P_gen [MW]/1
  pu to Hz2/1 -> ddtwg/1
  pu to Hz1/1 -> Omega/1
  pu to Hz/s/1 -> Omega_dot/1
  Gain2/1 -> Mux3/1
  Gain3/1 -> Mux3/2
  Mux7/1 -> To Workspace4/1
  State-Space/1 -> Mux7/4, pu to Hz2/1
  Mux/1 -> State-Space/1, Mux7/1, pu to Hz/1
